simulink model "myBERToolSim"  (Simulink 7.3)
settings: Solver=ode3  StartTime=0.0  StopTime=10  FixedStep=1/DataRate/xFd  RelTol=1e-3
values from neighbouring files (symbols this model uses):
  xFd = 8    [myBERTool.m]
undefined symbols (not defined in the file or in its folder): DataRate, EbNo
libraries: dspsnks4 x3, simulink x2, commutil2 x2, commfilt2 x1, commchan3 x1, commsink2 x1, dsparch4 x1, commrandsrc2 x1, dspstat3 x1, dspsrcs4 x1
settings Model: Creator=acarroll  LastModifiedBy=acarroll

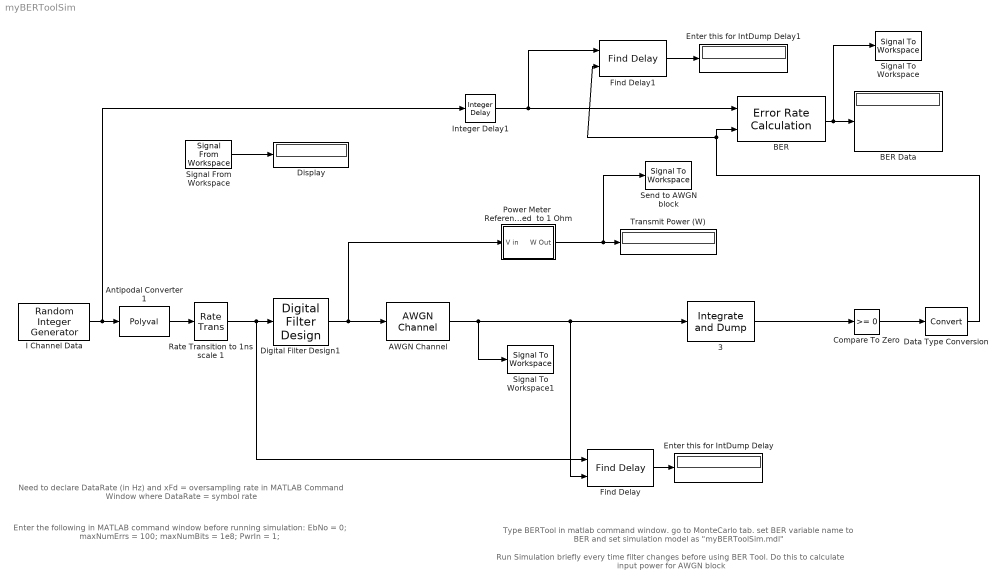
== system myBERToolSim ==
  note: Need to declare DataRate (in Hz)
      | and xFd = oversampling rate in MATLAB
      | Command Window where DataRate = symbol rate
  note: Enter the following in MATLAB command window before running simulation:
      | EbNo = 0; maxNumErrs = 100; maxNumBits = 1e8; PwrIn = 1;
  note: Run Simulation briefly every time filter changes before using BER Tool. Do this to calculate input power for AWGN block
  note: Type BERTool in matlab command window. go to MonteCarlo tab. set BER variable name to BER and set simulation model as "myBERToolSim.mdl"
  " 3" : commfilt2/Integrate and Dump  DialogController=commDDGCreate  DialogControllerArgs=DataTag0  obssamples=xFd  offsetsamples=6  nodump=off  roundingMode=Floor  overflowMode=off
  AWGN Channel : commchan3/AWGN Channel  SystemSampleTime=-1  seed=randseed  noiseMode="Signal to noise ratio  (Eb/No)"  EbNodB=EbNo  EsNodB=10  SNRdB=EbNo - 10*log10(xFd)  bitsPerSym=1  Ps=PwrIn  Tsym=1/DataRate  variance=0
  Antipodal Converter 1 : Polyval  Coefs=[ 2 -1 ]
  BER : commsink2/Error Rate Calculation  N=0  st_delay=20  cp_mode=Entire frame  subframe=[]  PMode=Port  WsName=ErrorVec  RsMode2=off  stop=on  numErr=maxNumErrs  maxBits=maxNumBits
  BER Data : Display
      settings: Format=short_e
  Compare To Zero : simulink/Logic and Bit Operations/Compare To Zero  SystemSampleTime=-1  relop=>=  LogicOutDataTypeMode=uint8  ZeroCross=off
  Data Type Conversion : DataTypeConversion  OutDataType=fixdt(1, 16)  OutScaling=2^0
  Digital Filter Design1 : dsparch4/Digital Filter Design  SystemSampleTime=-1  mwdsp_browser_bugfix_var=off
  Display : Display
  Enter this for IntDump Delay : Display
  Enter this for IntDump Delay1 : Display
  Find Delay : commutil2/Find Delay  SystemSampleTime=-1  corrLength=5000  chgSigOP=off  stopUpdate=off  numConstDelay=3
  Find Delay1 : commutil2/Find Delay  SystemSampleTime=-1  corrLength=50  chgSigOP=off  stopUpdate=off  numConstDelay=3
  I Channel Data : commrandsrc2/Random Integer Generator  SystemSampleTime=-1  mul=2  seed=randseed  Ts=1/DataRate  frameBased=off  sampPerFrame=50  orient=on  outDataType=double
  Integer Delay1 : simulink/Discrete/Integer Delay  vinit=0.0  samptime=-1  NumDelays=3
  Power Meter  Referenced  to 1 Ohm : Subsystem
  Rate Transition to 1ns scale 1 : RateTransition  OutPortSampleTime=1/DataRate/xFd
  Send to AWGN block : dspsnks4/Signal To Workspace  SystemSampleTime=-1  VariableName=PwrIn  FrameMode=Concatenate frames (2-D array)
      settings: MaxDataPoints=1  FixptAsFi=off
  Signal From Workspace : dspsrcs4/Signal From Workspace  SystemSampleTime=-1  X=EbNo  Ts=1  nsamps=1  OutputAfterFinalValue=Setting to zero  ignoreOrWarnInputAndFrameLengths=off
  Signal To Workspace : dspsnks4/Signal To Workspace  SystemSampleTime=-1  VariableName=BER  FrameMode=Concatenate frames (2-D array)
      settings: MaxDataPoints=1  FixptAsFi=off
  Signal To Workspace1 : dspsnks4/Signal To Workspace  SystemSampleTime=-1  VariableName=Test  FrameMode=Concatenate frames (2-D array)
      settings: MaxDataPoints=2^16  FixptAsFi=off
  Transmit Power (W) : Display
  wires:
  I Channel Data/1 -> Antipodal Converter 1/1, Integer Delay1/1
  Rate Transition to 1ns scale 1/1 -> Digital Filter Design1/1, Find Delay/1
  AWGN Channel/1 -> Signal To Workspace1/1, Find Delay/2, " 3"/1
  BER/1 -> BER Data/1, Signal To Workspace/1
  Power Meter  Referenced  to 1 Ohm/1(W Out) -> Transmit Power (W)/1, Send to AWGN block/1
  Signal From Workspace/1 -> Display/1
  " 3"/1 -> Compare To Zero/1
  Compare To Zero/1 -> Data Type Conversion/1
  Data Type Conversion/1 -> BER/2, Find Delay1/2
  Antipodal Converter 1/1 -> Rate Transition to 1ns scale 1/1
  Digital Filter Design1/1 -> Power Meter  Referenced  to 1 Ohm/1(V in), AWGN Channel/1
  Find Delay/1 -> Enter this for IntDump Delay/1
  Find Delay1/1 -> Enter this for IntDump Delay1/1
  Integer Delay1/1 -> BER/1, Find Delay1/1

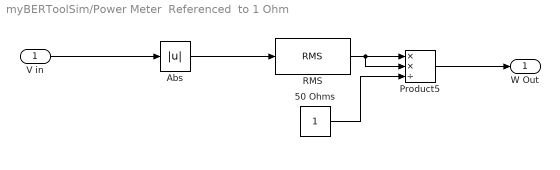
== system myBERToolSim/Power Meter  Referenced  to 1 Ohm ==
  V in : Inport
  50 Ohms : Constant  OutDataType=fixdt(1, 16)  OutScaling=2^0
  Abs : Abs  OutDataType=fixdt(1, 16)  OutScaling=2^0
  Product5 : Product  Inputs=**/  OutDataType=fixdt(1, 16)  OutScaling=2^0  RndMeth=Zero
  RMS : dspstat3/RMS  DialogController=dspDDGCreate  DialogControllerArgs=DataTag2  run=on  reset_popup=None  directionMode=Each column  dimension=1  treatSBRowAsCol=on
  W Out : Outport
  wires:
  50 Ohms/1 -> Product5/3
  RMS/1 -> Product5/2, Product5/1
  V in/1 -> Abs/1
  Product5/1 -> W Out/1
  Abs/1 -> RMS/1
